simulink model "KF_LQR_final"  (R2018b)
settings: Solver=VariableStepAuto  StartTime=0.0  StopTime=60  RelTol=1e-3
values from neighbouring files (symbols this model uses):
  Rv = diag([10^-2 10^-2])    [kf_test_2.m]    (also in kf_test_3.m; lab_init_lqr.m = diag([10^-5 10^-5]))
  x0 = [0 ... (first row only)    [kf_test_2.m]    (also in kf_test_3.m; lab_init_lqr.m)
undefined symbols (not defined in the file or in its folder): Continuous, Time
libraries: cstblocks x4, ctrlSharedLib x1
settings Model: Creator=prana  LastModifiedBy=ACSI-MLC

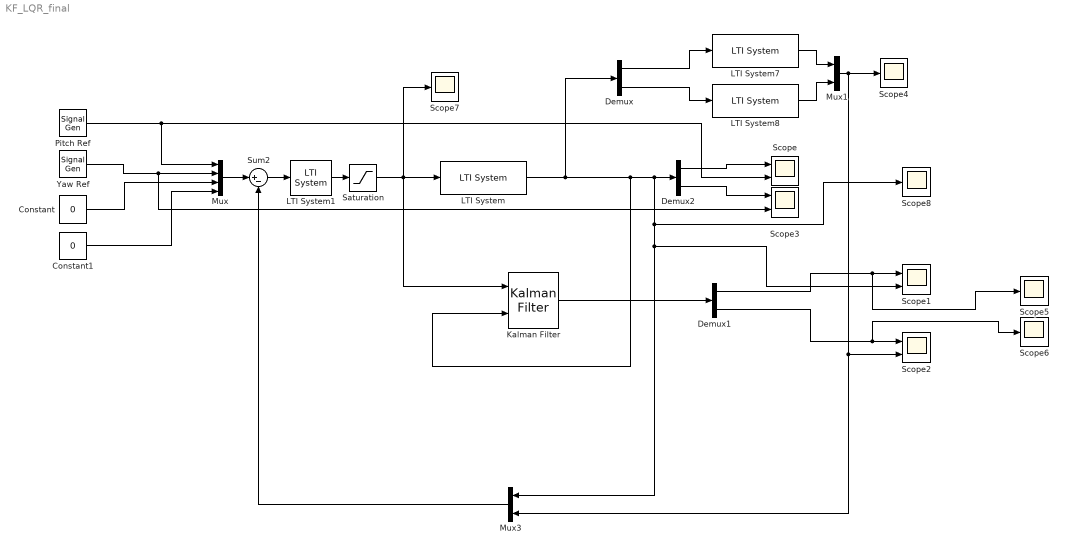
== system KF_LQR_final ==
  Constant : Constant  Value=0
  Constant1 : Constant  Value=0
  Demux : Demux  Outputs=2
  Demux1 : Demux  Outputs=2
  Demux2 : Demux  Outputs=2
  Kalman Filter : ctrlSharedLib/Kalman Filter  TimeDomain=Continuous-Time  UseCurrentEstimator=on  ModelSource=LTI State-Space Variable  ModelSourceVariable=aero_sys  A=0.95  B=1  C=1  D=0  NumberOfStates=1  NumberOfInputs=1  NumberOfOutputs=1  InitialEstimateSource=Dialog  X0=x0  P0=10  UseK=off  UseGH=off  NumberOfProcessNoiseInputs=1  G=1  TimeInvariantG=on  H=0  TimeInvariantH=on  Q=Rw  TimeInvariantQ=on  R=Rv  TimeInvariantR=on  N=0  TimeInvariantN=on  AddInputPort=on  AddEnablePort=off  OutputEstimatedY=off  OutputP=off  Ts=-1
      settings: SourceProductBaseCode=CT
  LTI System : cstblocks/LTI System  sys=aero_sys  IC=[]
  LTI System1 : cstblocks/LTI System  sys=K_lqr  IC=[]
  LTI System7 : cstblocks/LTI System  sys=Diff_LPF  IC=[]
  LTI System8 : cstblocks/LTI System  sys=Diff_LPF  IC=[]
  Mux : Mux
  Mux1 : Mux  Inputs=2
  Mux3 : Mux  Inputs=2
  Pitch Ref : SignalGenerator  WaveForm=square  Amplitude=pi/6  Frequency=0.4  Units=rad/sec
  Saturation : Saturate  UpperLimit=25  LowerLimit=-25
  Scope{,1..3} (4 alike) : Scope  NumInputPorts=2
  Scope{4..8} (5 alike) : Scope
  Sum2 : Sum  Inputs=|+-
  Yaw Ref : SignalGenerator  WaveForm=square  Amplitude=pi/4  Frequency=0.5  Units=rad/sec
  wires:
  Sum2/1 -> LTI System1/1
  Mux/1 -> Sum2/1
  Yaw Ref/1 -> Scope3/2, Mux/2
  Pitch Ref/1 -> Mux/1, Scope/2
  LTI System8/1 -> Mux1/2
  LTI System7/1 -> Mux1/1
  Demux/1 -> LTI System7/1
  Demux/2 -> LTI System8/1
  Constant/1 -> Mux/3
  Constant1/1 -> Mux/4
  Kalman Filter/1 -> Demux1/1
  Demux1/1 -> Scope5/1, Scope1/1
  Demux1/2 -> Scope6/1, Scope2/1
  LTI System1/1 -> Saturation/1
  Saturation/1 -> Kalman Filter/1, LTI System/1, Scope7/1
  Demux2/1 -> Scope/1
  Demux2/2 -> Scope3/1
  Mux3/1 -> Sum2/2
  LTI System/1 -> Demux/1, Scope8/1, Mux3/1, Scope1/2, Demux2/1, Kalman Filter/2
  Mux1/1 -> Mux3/2, Scope2/2, Scope4/1
